simulink model "csu_rtd_translational_dynamics_hrn"  (R2014b)
settings: Solver=FixedStepDiscrete  StartTime=0.0  StopTime=1  FixedStep=1  RelTol=1e-3
libraries: csu_rtd_translational_dynamics_lib x1, util_quat_lib x1
settings Model: Creator=hcannon  LastModifiedBy=mstewart
settings DataIOCC: SignalLoggingSaveFormat=ModelDataLogs
settings OptimizationCC: ExpressionDepthLimit=2147483647  InitFltsAndDblsToZero=on
settings DebuggingCC: UnderspecifiedInitializationDetection=Classic  MergeDetectMultiDrivingBlocksExec=none  FcnCallInpInsideContextMsg=UseLocalSettings  StateNameClashWarn=warning  StrictBusMsg=Warning
settings GRTTargetCC: CombineOutputUpdateFcns=off  GRTInterface=on

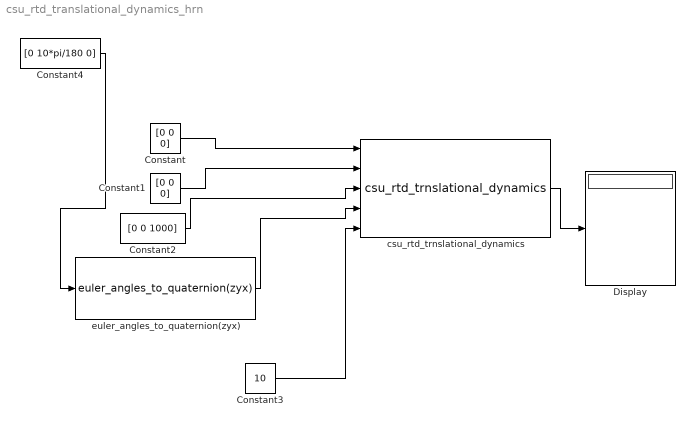
== system csu_rtd_translational_dynamics_hrn ==
  Constant : Constant  Value=[0 0 0]
  Constant1 : Constant  Value=[0 0 0]
  Constant2 : Constant  Value=[0 0 1000]
  Constant3 : Constant  Value=10
  Constant4 : Constant  Value=[0 10*pi/180 0]
  Display : Display
  csu_rtd_trnslational_dynamics : csu_rtd_translational_dynamics_lib/csu_rtd_trnslational_dynamics
  euler_angles_to_quaternion(zyx) : util_quat_lib/euler_angles_to_quaternion(zyx)  SystemSampleTime=-1
  wires:
  Constant/1 -> csu_rtd_trnslational_dynamics/1
  Constant1/1 -> csu_rtd_trnslational_dynamics/2
  Constant2/1 -> csu_rtd_trnslational_dynamics/3
  euler_angles_to_quaternion(zyx)/1 -> csu_rtd_trnslational_dynamics/4
  Constant3/1 -> csu_rtd_trnslational_dynamics/5
  Constant4/1 -> euler_angles_to_quaternion(zyx)/1
  csu_rtd_trnslational_dynamics/1 -> Display/1
